simulink model "Control_of_Grid_converter"  (R2020a)
settings: Solver=ode45  StartTime=0  StopTime=.1  MaxStep=Ts  RelTol=1e-3  AbsTol=1e-3  EnableMultiTasking=on
undefined symbols (not defined in the file or in its folder): alphac, C, Lf, pmax, Ts, ugN, w0_dc, w0_pll, wg
libraries: simulink x2
settings Model: Creator=mhinkkan  LastModifiedBy=yk_yo
settings SolverCC: AutoScaleAbsTol=off
settings DataIOCC: SaveFormat=Array  SignalLoggingSaveFormat=ModelDataLogs  SaveOutput=off  SignalLogging=off  DSMLogging=off  SaveTime=off  ReturnWorkspaceOutputs=off
settings OptimizationCC: BlockReduction=off  BooleanDataType=off  DefaultParameterBehavior=Inlined  OptimizeBlockIOStorage=off  BufferReuse=off  ExpressionFolding=off  ExpressionDepthLimit=2147483647  LocalBlockOutputs=off  InitFltsAndDblsToZero=on  LifeSpan=inf
settings DebuggingCC: SaveWithParameterizedLinksMsg=none  UnderspecifiedInitializationDetection=Classic  MergeDetectMultiDrivingBlocksExec=none  SignalResolutionControl=TryResolveAllWithWarning  MultiTaskDSMMsg=warning  MultiTaskCondExecSysMsg=none  FcnCallInpInsideContextMsg=warning  StateNameClashWarn=warning  SFUnexpectedBacktrackingDiag=warning  SFNoUnconditionalDefaultTransitionDiag=warning  SFExecutionAtInitializationDiag=none  ArithmeticOperatorsInVariantConditions=warning
settings HardwareCC: ProdBitPerPointer=32  ProdBitPerSizeT=32  ProdBitPerPtrDiffT=32  ProdLargestAtomicFloat=None  ProdIntDivRoundTo=Undefined  ProdEndianess=Unspecified  ProdWordSize=32  ProdHWDeviceType=32-bit Generic  TargetUnknown=on
settings ModelReferenceCC: PropagateSignalLabelsOutOfModel=off
settings SFSimCC: SimUseLocalCustomCode=off  CustomCodeUndefinedFunction=UseInterfaceOnly
settings RTWCC: RTWUseLocalCustomCode=off
settings CodeAppCC: StateflowObjectComments=on
settings GRTTargetCC: TargetFcnLib=ansi_tfl_tmw.mat  TargetLangStandard=C89/C90 (ANSI)  CombineOutputUpdateFcns=off  GRTInterface=on
settings ConfigComp: CovMetricSettings=dw  CovHtmlReporting=on  CovSaveCumulativeToWorkspaceVar=on  CovSaveSingleToWorkspaceVar=on  CovExternalEMLEnable=off

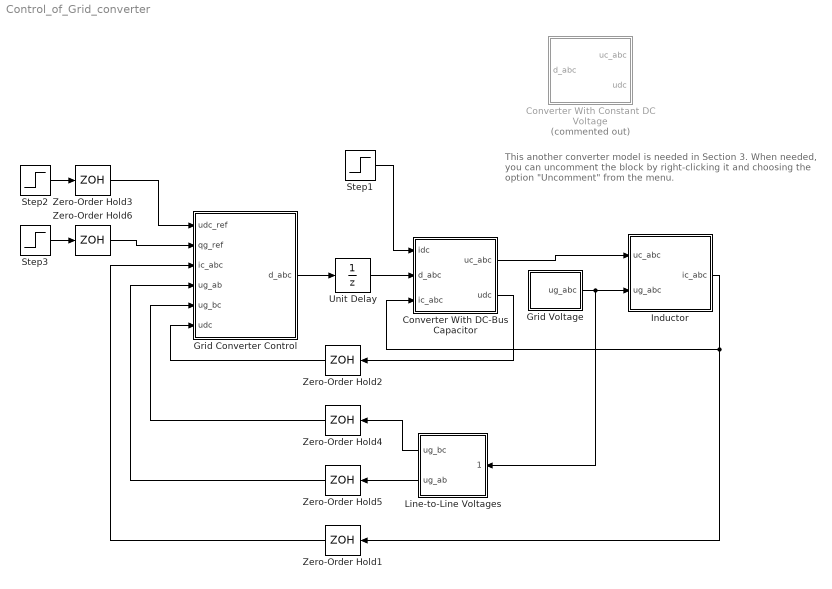
== system Control_of_Grid_converter ==
  note: This another converter model is needed in Section 3.
      | When needed, you can uncomment the block by right-clicking it
      | and choosing the option "Uncomment" from the menu.
  "Converter With Constant DC Voltage " : Subsystem  Commented=on  mask{fsw=8e3, Udc=650}
      mask prompts: fsw "Switching frequency (Hz)"; Udc "DC-bus voltage (V)"
      mask init:
      | Ts = 1/(2*fsw);
  Converter With DC-Bus Capacitor : Subsystem  mask{C=1e-3, fsw=8e3, udc0=600}
      mask prompts: C "DC-bus capacitance (F)"; fsw "Switching frequency (Hz)"; udc0 "Initial capacitor voltage (V)"
      mask init:
      | Ts = 1/(2*fsw);
  Grid Converter Control : Subsystem
  Grid Voltage : Subsystem  mask{wg=2*pi*50, Ug=400}
      mask prompts: wg "Grid angular frequency (rad/s)"; Ug "Line-line rms grid voltage (V)"
  Inductor : Subsystem  mask{Lf=10e-3, Rf=0}
      mask prompts: Lf "Inductance (H)"; Rf "Series resistance (ohm)"
  Line-to-Line Voltages : Subsystem
  Step1 : Step  Time=.06  After=10  SampleTime=0
  Step2 : Step  Time=0.02  Before=600  After=650  SampleTime=Ts
  Step3 : Step  Time=0.04  After=4e3  SampleTime=Ts
  Unit Delay : UnitDelay  SampleTime=Ts  HasFrameUpgradeWarning=on
  Zero-Order Hold{1..6} (6 alike) : ZeroOrderHold  SampleTime=Ts
  wires:
  Zero-Order Hold3/1 -> Grid Converter Control/1(udc_ref)
  Zero-Order Hold1/1 -> Grid Converter Control/3(ic_abc)
  Zero-Order Hold2/1 -> Grid Converter Control/6(udc)
  Step2/1 -> Zero-Order Hold3/1
  Zero-Order Hold4/1 -> Grid Converter Control/5(ug_bc)
  Zero-Order Hold5/1 -> Grid Converter Control/4(ug_ab)
  Grid Converter Control/1(d_abc) -> Unit Delay/1
  Step3/1 -> Zero-Order Hold6/1
  Zero-Order Hold6/1 -> Grid Converter Control/2(qg_ref)
  Inductor/1(ic_abc) -> Converter With DC-Bus Capacitor/3(ic_abc), Zero-Order Hold1/1
  Grid Voltage/1(ug_abc) -> Inductor/2(ug_abc), Line-to-Line Voltages/1(ug_abc)
  Line-to-Line Voltages/1(ug_bc) -> Zero-Order Hold4/1
  Line-to-Line Voltages/2(ug_ab) -> Zero-Order Hold5/1
  Step1/1 -> Converter With DC-Bus Capacitor/1(idc)
  Unit Delay/1 -> Converter With DC-Bus Capacitor/2(d_abc)
  Converter With DC-Bus Capacitor/1(uc_abc) -> Inductor/1(uc_abc)
  Converter With DC-Bus Capacitor/2(udc) -> Zero-Order Hold2/1

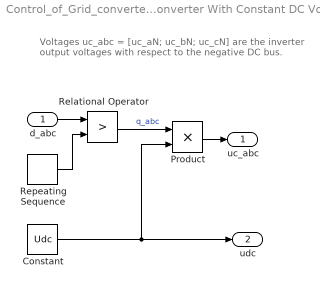
== system Control_of_Grid_converter/Converter With Constant DC Voltage  ==
  note: Voltages uc_abc = [uc_aN; uc_bN; uc_cN] are the inverter
      | output voltages with respect to the negative DC bus.
  d_abc : Inport
  Constant : Constant  Value=Udc
  Product : Product
  Relational Operator : RelationalOperator  Operator=>  OutDataTypeStr='double'  RndMeth=Nearest
  Repeating Sequence : simulink/Sources/Repeating Sequence  rep_seq_t=[0 1 2]*Ts  rep_seq_y=[1 0 1]
  uc_abc : Outport
  udc : Outport  Port=2
  wires:
  Repeating Sequence/1 -> Relational Operator/2
  d_abc/1 -> Relational Operator/1
  Product/1 -> uc_abc/1
  Relational Operator/1 -> Product/1  "q_abc"
  Constant/1 -> Product/2, udc/1

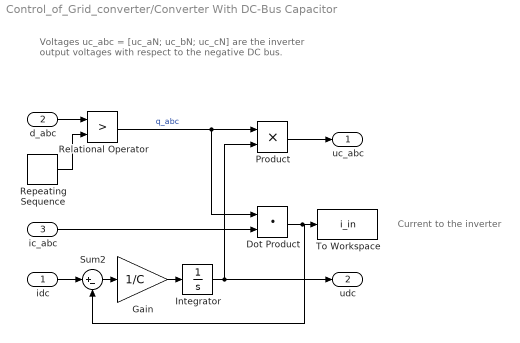
== system Control_of_Grid_converter/Converter With DC-Bus Capacitor ==
  note: Current to the inverter
  note: Voltages uc_abc = [uc_aN; uc_bN; uc_cN] are the inverter
      | output voltages with respect to the negative DC bus.
  idc : Inport
  d_abc : Inport  Port=2
  ic_abc : Inport  Port=3
  Dot Product : DotProduct  InputSameDT=on  OutDataTypeStr=Inherit: Inherit via internal rule
  Gain : Gain  Gain=1/C
  Integrator : Integrator  InitialCondition=udc0
  Product : Product
  Relational Operator : RelationalOperator  Operator=>  OutDataTypeStr='double'  RndMeth=Nearest
  Repeating Sequence : simulink/Sources/Repeating Sequence  rep_seq_t=[0 1 2]*Ts  rep_seq_y=[1 0 1]
  Sum2 : Sum  Inputs=|+-
  To Workspace : ToWorkspace  VariableName=i_in  SaveFormat=Timeseries  SampleTime=-1
  uc_abc : Outport
  udc : Outport  Port=2
  wires:
  Repeating Sequence/1 -> Relational Operator/2
  d_abc/1 -> Relational Operator/1
  Sum2/1 -> Gain/1
  Gain/1 -> Integrator/1
  idc/1 -> Sum2/1
  Dot Product/1 -> Sum2/2, To Workspace/1
  Integrator/1 -> Product/2, udc/1
  Product/1 -> uc_abc/1
  Relational Operator/1 -> Dot Product/1, Product/1  "q_abc"
  ic_abc/1 -> Dot Product/2

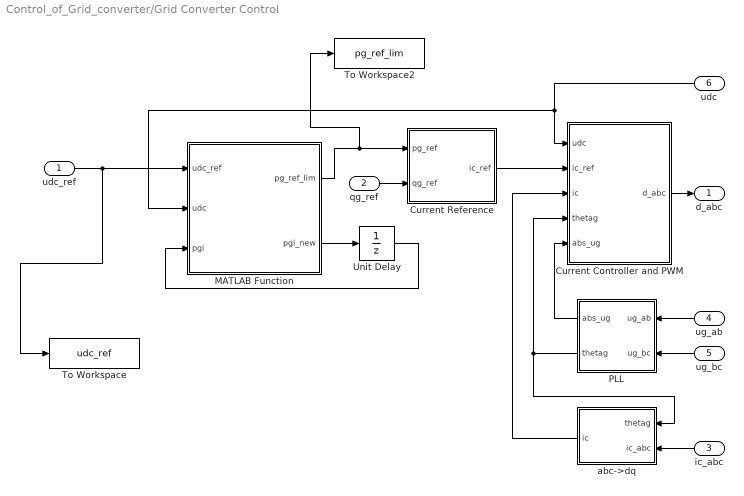
== system Control_of_Grid_converter/Grid Converter Control ==
  udc_ref : Inport
  qg_ref : Inport  Port=2
  ic_abc : Inport  Port=3
  ug_ab : Inport  Port=4
  ug_bc : Inport  Port=5
  udc : Inport  Port=6
  Current Controller and PWM : Subsystem
  Current Reference : Subsystem
  MATLAB Function : MATLAB Function  TreatAsAtomicUnit=on
  PLL : Subsystem
  To Workspace : ToWorkspace  VariableName=udc_ref  SaveFormat=Timeseries  SampleTime=-1
  To Workspace2 : ToWorkspace  VariableName=pg_ref_lim  SaveFormat=Timeseries  SampleTime=-1
  Unit Delay : UnitDelay  InitialCondition=wg  SampleTime=-1  HasFrameUpgradeWarning=on
  abc->dq : Subsystem
  d_abc : Outport
  wires:
  ic_abc/1 -> abc->dq/2(ic_abc)
  Current Controller and PWM/1(d_abc) -> d_abc/1
  Current Reference/1(ic_ref) -> Current Controller and PWM/2(ic_ref)
  abc->dq/1(ic) -> Current Controller and PWM/3(ic)
  qg_ref/1 -> Current Reference/2(qg_ref)
  ug_bc/1 -> PLL/2(ug_bc)
  ug_ab/1 -> PLL/1(ug_ab)
  PLL/2(thetag) -> abc->dq/1(thetag), Current Controller and PWM/4(thetag)
  udc/1 -> MATLAB Function/2(udc), Current Controller and PWM/1(udc)
  udc_ref/1 -> To Workspace/1, MATLAB Function/1(udc_ref)
  MATLAB Function/1(pg_ref_lim) -> To Workspace2/1, Current Reference/1(pg_ref)
  MATLAB Function/2(pgi_new) -> Unit Delay/1
  Unit Delay/1 -> MATLAB Function/3(pgi)
  PLL/1(abs_ug) -> Current Controller and PWM/5(abs_ug)

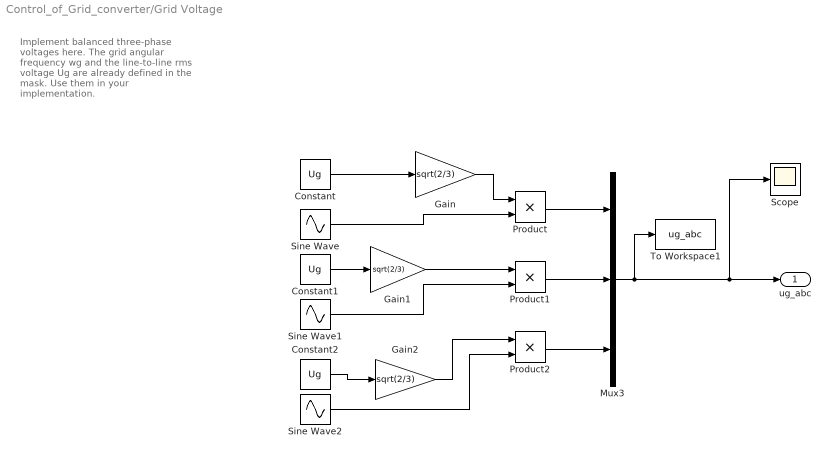
== system Control_of_Grid_converter/Grid Voltage ==
  note: Implement balanced three-phase
      | voltages here. The grid angular
      | frequency wg and the line-to-line rms
      | voltage Ug are already defined
      | in the mask. Use them in your
      | implementation.
  Constant : Constant  Value=Ug
  Constant1 : Constant  Value=Ug
  Constant2 : Constant  Value=Ug
  Gain : Gain  Gain=sqrt(2/3)
  Gain1 : Gain  Gain=sqrt(2/3)
  Gain2 : Gain  Gain=sqrt(2/3)
  Mux3 : Mux  Inputs=3
  Product : Product
  Product1 : Product
  Product2 : Product
  Scope : Scope
  Sine Wave : Sin  Frequency=wg  Phase=pi/2  SampleTime=0
  Sine Wave1 : Sin  Frequency=wg  Phase=(pi/2)-(2*pi/3)  SampleTime=0
  Sine Wave2 : Sin  Frequency=wg  Phase=(pi/2)-(4*pi/3)  SampleTime=0
  To Workspace1 : ToWorkspace  VariableName=ug_abc  SaveFormat=Timeseries  SampleTime=-1
  ug_abc : Outport
  wires:
  Mux3/1 -> To Workspace1/1, Scope/1, ug_abc/1
  Product/1 -> Mux3/1
  Product2/1 -> Mux3/3
  Product1/1 -> Mux3/2
  Sine Wave/1 -> Product/2
  Sine Wave1/1 -> Product1/2
  Sine Wave2/1 -> Product2/2
  Constant/1 -> Gain/1
  Gain/1 -> Product/1
  Constant1/1 -> Gain1/1
  Gain1/1 -> Product1/1
  Constant2/1 -> Gain2/1
  Gain2/1 -> Product2/1

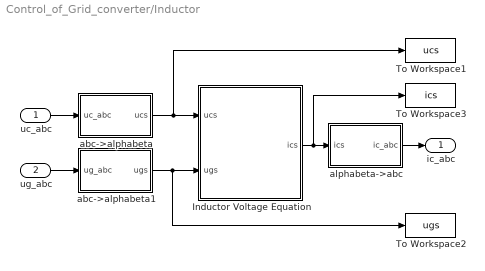
== system Control_of_Grid_converter/Inductor ==
  uc_abc : Inport
  ug_abc : Inport  Port=2
  Inductor Voltage Equation : Subsystem
  To Workspace1 : ToWorkspace  VariableName=ucs  SaveFormat=Timeseries
  To Workspace2 : ToWorkspace  VariableName=ugs  SaveFormat=Timeseries
  To Workspace3 : ToWorkspace  VariableName=ics  SaveFormat=Timeseries
  abc->alphabeta : Subsystem
  abc->alphabeta1 : Subsystem
  alphabeta->abc : Subsystem
  ic_abc : Outport
  wires:
  uc_abc/1 -> abc->alphabeta/1(uc_abc)
  Inductor Voltage Equation/1(ics) -> To Workspace3/1, alphabeta->abc/1(ics)
  abc->alphabeta/1(ucs) -> To Workspace1/1, Inductor Voltage Equation/1(ucs)
  alphabeta->abc/1(ic_abc) -> ic_abc/1
  ug_abc/1 -> abc->alphabeta1/1(ug_abc)
  abc->alphabeta1/1(ugs) -> To Workspace2/1, Inductor Voltage Equation/2(ugs)

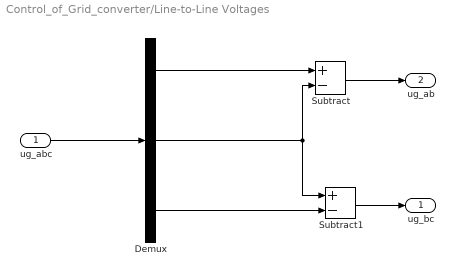
== system Control_of_Grid_converter/Line-to-Line Voltages ==
  ug_abc : Inport
  Demux : Demux  Outputs=3
  Subtract : Sum  Inputs=+-
  Subtract1 : Sum  Inputs=+-
  ug_bc : Outport
  ug_ab : Outport  Port=2
  wires:
  ug_abc/1 -> Demux/1
  Demux/1 -> Subtract/1
  Subtract/1 -> ug_ab/1
  Demux/3 -> Subtract1/2
  Subtract1/1 -> ug_bc/1
  Demux/2 -> Subtract/2, Subtract1/1

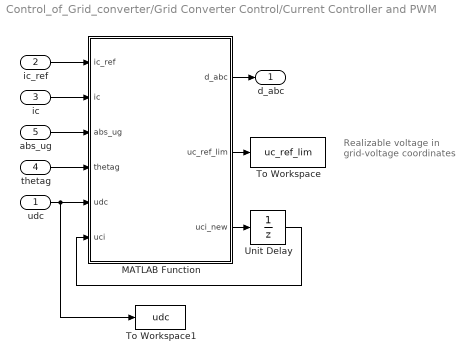
== system Control_of_Grid_converter/Grid Converter Control/Current Controller and PWM ==
  note: Realizable voltage
      | in grid-voltage coordinates
  udc : Inport
  ic_ref : Inport  Port=2
  ic : Inport  Port=3
  thetag : Inport  Port=4
  abs_ug : Inport  Port=5
  MATLAB Function : MATLAB Function  TreatAsAtomicUnit=on
  To Workspace : ToWorkspace  VariableName=uc_ref_lim  SaveFormat=Timeseries  SampleTime=-1
  To Workspace1 : ToWorkspace  VariableName=udc  SaveFormat=Timeseries  SampleTime=-1
  Unit Delay : UnitDelay  SampleTime=-1  HasFrameUpgradeWarning=on
  d_abc : Outport  PortDimensions=3
  wires:
  MATLAB Function/3(uci_new) -> Unit Delay/1
  ic_ref/1 -> MATLAB Function/1(ic_ref)
  ic/1 -> MATLAB Function/2(ic)
  Unit Delay/1 -> MATLAB Function/6(uci)
  MATLAB Function/1(d_abc) -> d_abc/1
  MATLAB Function/2(uc_ref_lim) -> To Workspace/1
  thetag/1 -> MATLAB Function/4(thetag)
  udc/1 -> To Workspace1/1, MATLAB Function/5(udc)
  abs_ug/1 -> MATLAB Function/3(abs_ug)

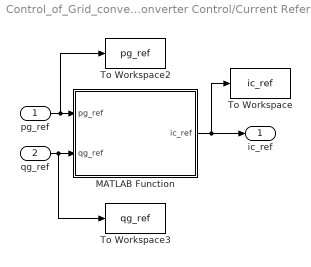
== system Control_of_Grid_converter/Grid Converter Control/Current Reference ==
  pg_ref : Inport
  qg_ref : Inport  Port=2
  MATLAB Function : MATLAB Function  TreatAsAtomicUnit=on
  To Workspace : ToWorkspace  VariableName=ic_ref  SaveFormat=Timeseries  SampleTime=-1
  To Workspace2 : ToWorkspace  VariableName=pg_ref  SaveFormat=Timeseries  SampleTime=-1
  To Workspace3 : ToWorkspace  VariableName=qg_ref  SaveFormat=Timeseries  SampleTime=-1
  ic_ref : Outport
  wires:
  pg_ref/1 -> To Workspace2/1, MATLAB Function/1(pg_ref)
  MATLAB Function/1(ic_ref) -> To Workspace/1, ic_ref/1
  qg_ref/1 -> To Workspace3/1, MATLAB Function/2(qg_ref)

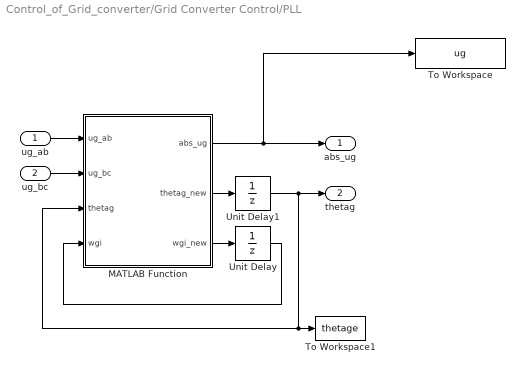
== system Control_of_Grid_converter/Grid Converter Control/PLL ==
  ug_ab : Inport
  ug_bc : Inport  Port=2
  MATLAB Function : MATLAB Function  TreatAsAtomicUnit=on
  To Workspace : ToWorkspace  VariableName=ug  SaveFormat=Timeseries  SampleTime=-1
  To Workspace1 : ToWorkspace  VariableName=thetage  SaveFormat=Timeseries  SampleTime=-1
  Unit Delay : UnitDelay  InitialCondition=wg  SampleTime=-1  HasFrameUpgradeWarning=on
  Unit Delay1 : UnitDelay  SampleTime=-1  HasFrameUpgradeWarning=on
  abs_ug : Outport
  thetag : Outport  Port=2
  wires:
  ug_bc/1 -> MATLAB Function/2(ug_bc)
  ug_ab/1 -> MATLAB Function/1(ug_ab)
  MATLAB Function/1(abs_ug) -> To Workspace/1, abs_ug/1
  MATLAB Function/3(wgi_new) -> Unit Delay/1
  MATLAB Function/2(thetag_new) -> Unit Delay1/1
  Unit Delay1/1 -> MATLAB Function/3(thetag), To Workspace1/1, thetag/1
  Unit Delay/1 -> MATLAB Function/4(wgi)

== system Control_of_Grid_converter/Grid Converter Control/abc->dq ==
  thetag : Inport
  ic_abc : Inport  Port=2
  MATLAB Function : MATLAB Function  TreatAsAtomicUnit=on
  To Workspace : ToWorkspace  VariableName=ic_abc  SaveFormat=Timeseries  SampleTime=-1
  To Workspace4 : ToWorkspace  VariableName=ic  SaveFormat=Timeseries  SampleTime=-1
  ic : Outport
  wires:
  MATLAB Function/1(ic) -> To Workspace4/1, ic/1
  thetag/1 -> MATLAB Function/2(thetag)
  ic_abc/1 -> To Workspace/1, MATLAB Function/1(ic_abc)

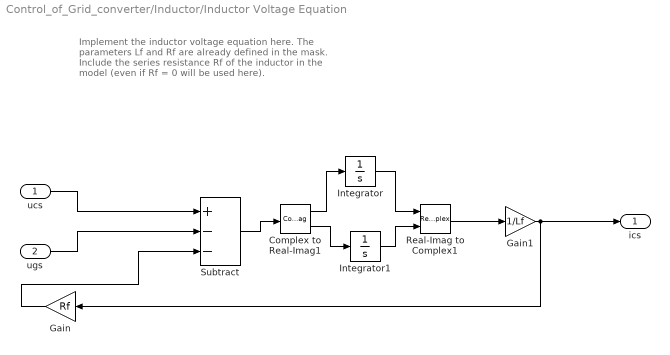
== system Control_of_Grid_converter/Inductor/Inductor Voltage Equation ==
  note: Implement the inductor voltage equation here.
      | The parameters Lf and Rf are already defined in the
      | mask. Include the series resistance Rf of the inductor
      | in the model (even if Rf = 0 will be used here).
  ucs : Inport
  ugs : Inport  Port=2
  Complex to Real-Imag1 : ComplexToRealImag
  Gain : Gain  Gain=Rf
  Gain1 : Gain  Gain=1/Lf
  Integrator : Integrator
  Integrator1 : Integrator
  Real-Imag to Complex1 : RealImagToComplex
  Subtract : Sum  Inputs=+--
  ics : Outport
  wires:
  Subtract/1 -> Complex to Real-Imag1/1
  Complex to Real-Imag1/1 -> Integrator/1
  Complex to Real-Imag1/2 -> Integrator1/1
  ugs/1 -> Subtract/2
  ucs/1 -> Subtract/1
  Gain/1 -> Subtract/3
  Integrator/1 -> Real-Imag to Complex1/1
  Integrator1/1 -> Real-Imag to Complex1/2
  Real-Imag to Complex1/1 -> Gain1/1
  Gain1/1 -> Gain/1, ics/1

== system Control_of_Grid_converter/Inductor/abc->alphabeta ==
  uc_abc : Inport
  Fcn : Fcn  Expr=2/3*(u(1)-0.5*u(2)-0.5*u(3))
  Fcn1 : Fcn  Expr=sqrt(3)/3*(u(2)-u(3))
  Real-Imag to Complex : RealImagToComplex
  ucs : Outport
  wires:
  uc_abc/1 -> Fcn1/1, Fcn/1
  Fcn/1 -> Real-Imag to Complex/1  "alpha"
  Fcn1/1 -> Real-Imag to Complex/2  "beta"
  Real-Imag to Complex/1 -> ucs/1

== system Control_of_Grid_converter/Inductor/abc->alphabeta1 ==
  ug_abc : Inport
  Fcn : Fcn  Expr=2/3*(u(1)-0.5*u(2)-0.5*u(3))
  Fcn1 : Fcn  Expr=sqrt(3)/3*(u(2)-u(3))
  Real-Imag to Complex : RealImagToComplex
  ugs : Outport
  wires:
  ug_abc/1 -> Fcn1/1, Fcn/1
  Fcn/1 -> Real-Imag to Complex/1  "alpha"
  Fcn1/1 -> Real-Imag to Complex/2  "beta"
  Real-Imag to Complex/1 -> ugs/1

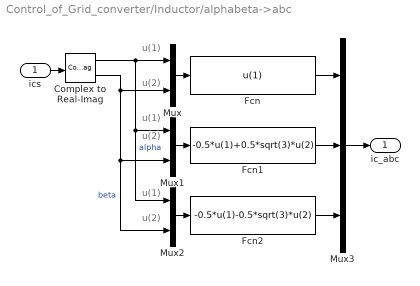
== system Control_of_Grid_converter/Inductor/alphabeta->abc ==
  note: u(1)
  note: u(2)
  note: u(1)
  note: u(2)
  note: u(1)
  note: u(2)
  ics : Inport
  Complex to Real-Imag : ComplexToRealImag
  Fcn : Fcn  Expr=u(1)
  Fcn1 : Fcn  Expr=-0.5*u(1)+0.5*sqrt(3)*u(2)
  Fcn2 : Fcn  Expr=-0.5*u(1)-0.5*sqrt(3)*u(2)
  Mux : Mux  Inputs=2
  Mux1 : Mux  Inputs=2
  Mux2 : Mux  Inputs=2
  Mux3 : Mux  Inputs=3
  ic_abc : Outport
  wires:
  Mux/1 -> Fcn/1
  Complex to Real-Imag/1 -> Mux/1, Mux1/1, Mux2/1  "alpha"
  Complex to Real-Imag/2 -> Mux/2, Mux1/2, Mux2/2  "beta"
  Mux1/1 -> Fcn1/1
  Mux2/1 -> Fcn2/1
  ics/1 -> Complex to Real-Imag/1
  Fcn/1 -> Mux3/1
  Fcn1/1 -> Mux3/2
  Fcn2/1 -> Mux3/3
  Mux3/1 -> ic_abc/1

== matlab function Control_of_Grid_converter/Grid Converter Control/Current Controller and PWM/MATLAB Function ==
  data: ic_ref input size=1; ic input size=1; abs_ug input; thetag input size=1; udc input size=1; uci input size=1; wg parameter; Lf parameter size=1; alphac parameter size=1; Ts parameter size=1; d_abc output size=3; uc_ref_lim output; uci_new output
function [d_abc, uc_ref_lim, uci_new] = cc(ic_ref,ic,abs_ug,thetag,udc,uci,wg,Lf,alphac,Ts)
%#codegen

%% Current controller 
% Gains
kp = alphac*Lf;
ki = alphac^2*Lf;
r = alphac*Lf;

% Voltage reference in synchronous coordinates
e = ic_ref - ic;
uc_ref = kp*e + uci - r*ic + 1j*wg*Lf*ic + abs_ug;

% Reference in stator coordinates
thetagc = thetag + 1.5*Ts*wg;   % Compensation for discrete-time delays
ucs_ref = uc_ref*exp(1j*thetagc);

%% Symmetrical suboscillation PWM
% Components of the voltage space vector
uc_alpha_ref = real(ucs_ref);
uc_beta_ref  = imag(ucs_ref);

% Phase-voltage references
uca_ref = uc_alpha_ref;
ucb_ref = .5*(-uc_alpha_ref + sqrt(3)*uc_beta_ref);
ucc_ref = .5*(-uc_alpha_ref - sqrt(3)*uc_beta_ref);

% Vector of phase-voltage references
uc_abc_ref = [uca_ref; ucb_ref; ucc_ref];

% Symmetrization of the references by adding the zero-sequence voltage
u0 = .5*(max(uc_abc_ref) + min(uc_abc_ref));
uc_abc_ref = uc_abc_ref - u0;

% Clipping of the reference voltages such that no phase error is caused. 
% If all phase voltage reference are realizable (below Udc/2), m = 1 holds.
m = max([2*uc_abc_ref/udc; 1]);
uc_abc_ref = uc_abc_ref/m;

% Duty cycles, which can be directly used for triangle comparison, 
% if the triangle wave varies between 0...1
d_abc = .5 + uc_abc_ref/udc;

% Realized voltage vector is calculated from the clamped duty ratios.
% If the PWM does not saturate, us_ref_lim = us_ref holds. The realized
% voltage vector is needed, e.g., for the current-controller antiwindup.
ucs_ref_lim = 2/3*(d_abc(1) + d_abc(2)*exp(1j*2*pi/3) + d_abc(3)*exp(1j*4*pi/3))*udc;
% In estimated rotor flux coordinates
uc_ref_lim = exp(-1j*thetagc)*ucs_ref_lim;  

%% Update the integral state of the current controller 
uci_new = uci + Ts*ki*(e + (uc_ref_lim - uc_ref)/kp);

== matlab function Control_of_Grid_converter/Grid Converter Control/PLL/MATLAB Function ==
  data: ug_ab input size=1; ug_bc input size=1; thetag input; wgi input; ugN parameter; w0_pll parameter; abs_ug output size=1; thetag_new output; wgi_new output; Ts parameter
function [abs_ug,thetag_new,wgi_new] = pll(ug_ab,ug_bc,thetag,wgi,ugN,w0_pll,Ts)
%#codegen

% Parameters 
% (Tuning of the PLL is analogous to that of the DC-voltage controller.)
zeta = 1;   % Damping ratio
kp = 2*zeta*w0_pll/ugN; 
ki = w0_pll^2/ugN;

% Space-vector transformation from line-to-line components
ugs = (2/3)*(ug_ab - (ug_bc*exp(1j*4*pi/3)))  ;  % Complete this

% Coordinate transformation to "estimated" grid-voltage coordinates
ug = ugs*exp(-1j*thetag);    % Complete this

% Error signal, which is drive to zero by the PLL
ugq = imag(ug); 	% Complete this

wg = kp*ugq + wgi;

% Update the integrator state
wgi_new = wgi + Ts*ki*ugq;

% Update the grid-voltage angle
thetag_new = thetag + Ts*wg;
while(thetag_new > pi)
    thetag_new = thetag_new - 2*pi;
end
while(thetag_new < -pi)
    thetag_new = thetag_new + 2*pi;
end

% Absolute value of the grid-voltage vector
abs_ug = abs(ug);

== matlab function Control_of_Grid_converter/Grid Converter Control/Current Reference/MATLAB Function ==
  data: pg_ref input; qg_ref input; ic_ref output; ugN parameter size=1
function ic_ref = curr_ref(pg_ref,qg_ref,ugN)
%#codegen

% Current references in grid-voltage coordinates
ic_ref = ((2*pg_ref)/(3*ugN))  -  ((1j*2*qg_ref)/(3*ugN))  % Complete this

== matlab function Control_of_Grid_converter/Grid Converter Control/abc->dq/MATLAB Function ==
  data: ic_abc input size=3; thetag input size=1; ic output size=1
function ic = abc_dq(ic_abc, thetag)
%#codegen

% Space-vector transformation
ics = 2/3*(ic_abc(1) + ic_abc(2)*exp(1j*2*pi/3) + ic_abc(3)*exp(1j*4*pi/3));
% Coordinate transformation
ic = ics*exp(-1j*thetag);

== matlab function Control_of_Grid_converter/Grid Converter Control/MATLAB Function ==
  data: udc_ref input; pg_ref_lim output; udc input; pgi input; C parameter size=1; pgi_new output; w0_dc parameter size=1; pmax parameter size=1; Ts parameter size=1
function [pg_ref_lim,pgi_new] = dcbus(udc_ref,udc,pgi,C, w0_dc, pmax, Ts)
%#codegen

% Gains (see Exercise 4)
zeta = 1;
kp = 2*zeta*w0_dc;
ki = w0_dc^2;

% Error signal (the capacitor energy)
e = (C/2) * (udc_ref^2 - udc^2) ; % Complete this

% PI controller
pg_ref = -kp*e - pgi;

% Limit the output reference
pg_ref_lim = pg_ref;
if(pg_ref_lim > pmax)
pg_ref_lim = pmax;
elseif(pg_ref_lim < -pmax)
pg_ref_lim = -pmax;
end

% Update the integrator state (the last term is anti-windup)
pgi_new = pgi + Ts*ki*(e + (pg_ref_lim - pg_ref)/kp);
